simulink model "zad333e_Sim"  (Simulink 7.1)
settings: Solver=ode45  StartTime=0.0  StopTime=10.0  RelTol=1e-3
settings Model: Creator=mestar  LastModifiedBy=mestar
settings DebuggingCC: SaveWithParameterizedLinksMsg=none  SignalResolutionControl=TryResolveAllWithWarning  MultiTaskDSMMsg=warning  MultiTaskCondExecSysMsg=none
settings RTWCC: IncludeERTFirstTime=on
settings GRTTargetCC: TargetFcnLib=ansi_tfl_tmw.mat

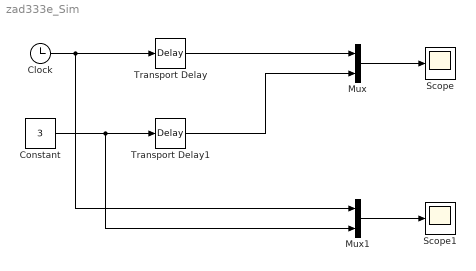
== system zad333e_Sim ==
  Clock : Clock
      settings: Decimation=10
  Constant : Constant  Value=3  OutDataType=sfix(16)  OutScaling=2^0
  Mux : Mux  Inputs=2
  Mux1 : Mux  Inputs=2
  Scope : Scope
  Scope1 : Scope
  Transport Delay : TransportDelay  DelayTime=2
  Transport Delay1 : TransportDelay  DelayTime=2
  wires:
  Mux/1 -> Scope/1
  Mux1/1 -> Scope1/1
  Clock/1 -> Transport Delay/1, Mux1/1
  Constant/1 -> Transport Delay1/1, Mux1/2
  Transport Delay/1 -> Mux/1
  Transport Delay1/1 -> Mux/2
